simulink model "tut3"  (R2025b)
settings: Solver=VariableStepAuto  StartTime=0.0  StopTime=10.0  RelTol=1e-3
values from neighbouring files (symbols this model uses):
  A = [0 1 0 0 ... (first row only)    [untitled2.m]    (also in untitled3.m)
  A_hat = A_bb - Ke*A_ab    [untitled2.m]
  Aref = 0.8    [untitled3.m]
  B = [0; 0; 0; 1/m2]    [untitled2.m]    (also in untitled3.m = [0;1/m1;0;0])
  B_hat = A_hat*Ke + A_ba - Ke*A_aa    [untitled2.m]
  c1 = 2    [untitled2.m]    (also in untitled3.m)
  c2 = 5    [untitled2.m]    (also in untitled3.m)
  C_hat = [zeros(1, 3) ... (first row only)    [untitled2.m]
  D_hat = [1 ... (first row only)    [untitled2.m]
  F_hat = B_b - Ke*B_a    [untitled2.m]
  k1 = 4    [untitled2.m]    (also in untitled3.m)
  k2 = 12    [untitled2.m]    (also in untitled3.m)
  Kd = 35    [untitled3.m]
  Ke = place(A_bb', A_ab', p_o)'    [untitled2.m]
  Ki = 10    [untitled3.m]
  Kp = 120    [untitled3.m]
  m1 = 3    [untitled2.m]    (also in untitled3.m)
  w = 2*pi*1    (= 6.28318530718)    [untitled3.m]
  z0 = [2; 1.5; 1]    [untitled2.m]
settings Model: Creator=Abhi  LastModifiedBy=Abhi

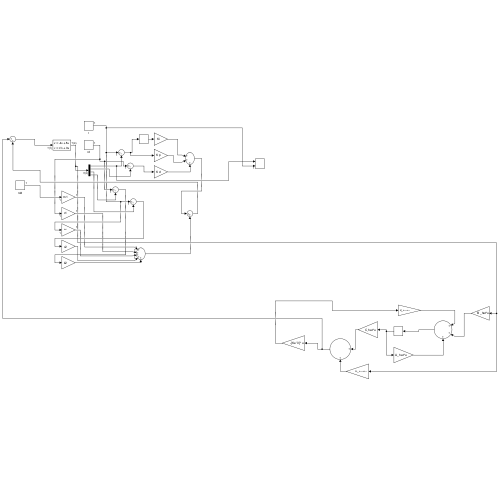
[thumbnail: Simulink's stored preview of the top-level diagram]
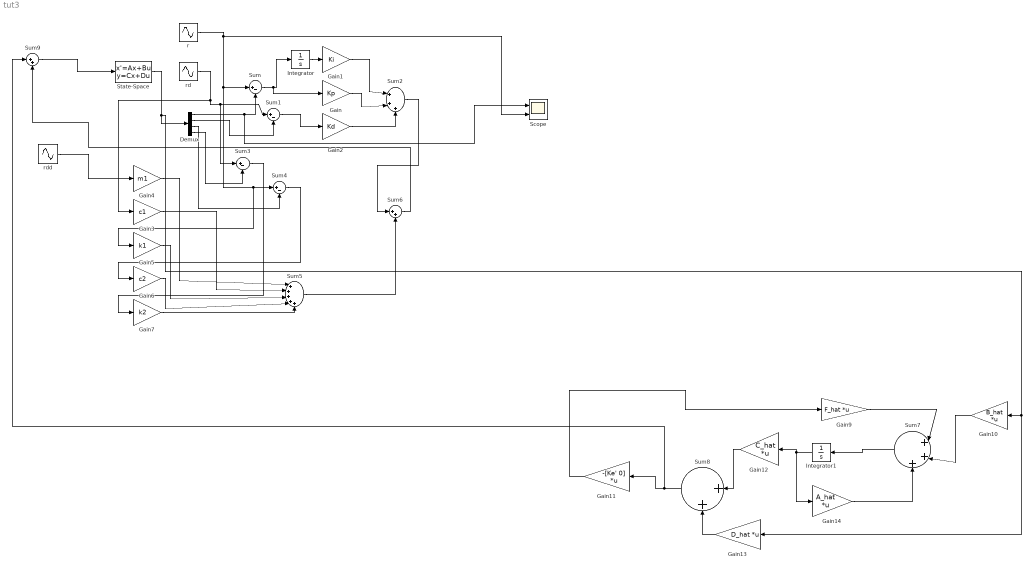
== system tut3 ==
  Demux : Demux
  Gain : Gain  Gain=Kp
  Gain1 : Gain  Gain=Ki
  Gain10 : Gain  Gain=B_hat  Multiplication=Matrix(K*u)
  Gain11 : Gain  Gain=-[Ke' 0]  Multiplication=Matrix(K*u)
  Gain12 : Gain  Gain=C_hat  Multiplication=Matrix(K*u)
  Gain13 : Gain  Gain=D_hat  Multiplication=Matrix(K*u)
  Gain14 : Gain  Gain=A_hat  Multiplication=Matrix(K*u)
  Gain2 : Gain  Gain=Kd
  Gain3 : Gain  Gain=c1
  Gain4 : Gain  Gain=m1
  Gain5 : Gain  Gain=k1
  Gain6 : Gain  Gain=c2
  Gain7 : Gain  Gain=k2
  Gain9 : Gain  Gain=F_hat  Multiplication=Matrix(K*u)
  Integrator : Integrator
  Integrator1 : Integrator  InitialCondition=z0
  Scope : Scope  NumInputPorts=2
      settings: ActiveDisplayYMinimum=-1.16819116268996  ActiveDisplayYMaximum=1.1667330676781473
  State-Space : StateSpace  A=A  B=B  C=eye(4)  D=zeros(4,1)  InitialCondition=[0.3 0.01 0 0]'
  Sum{,1,3..4} (4 alike) : Sum  Inputs=|+-
  Sum2 : Sum  Inputs=|+++
  Sum5 : Sum  Inputs=|+++++
  Sum6 : Sum  Inputs=|++
  Sum7 : Sum  Inputs=|+++
  Sum8 : Sum  Inputs=|++
  Sum9 : Sum  Inputs=|++
  r : Sin  Amplitude=Aref  Frequency=w  SampleTime=0
  rd : Sin  Amplitude=Aref*w  Frequency=w  Phase=pi/2  SampleTime=0
  rdd : Sin  Amplitude=Aref*w*w  Frequency=w  Phase=pi  SampleTime=0
  wires:
  Demux/1 -> Scope/1, Sum/2
  r/1 -> Scope/2, Gain5/1, Sum4/1, Sum/1
  Sum/1 -> Gain/1, Integrator/1
  Demux/2 -> Sum1/2
  rd/1 -> Gain3/1, Sum3/1, Sum1/1
  Integrator/1 -> Gain1/1
  Sum1/1 -> Gain2/1
  Gain1/1 -> Sum2/1
  Gain/1 -> Sum2/2
  Gain2/1 -> Sum2/3
  Demux/4 -> Sum3/2
  Demux/3 -> Sum4/2
  rdd/1 -> Gain4/1
  Sum3/1 -> Gain7/1
  Sum4/1 -> Gain6/1
  Gain4/1 -> Sum5/1
  Gain3/1 -> Sum5/2
  Gain5/1 -> Sum5/3
  Gain6/1 -> Sum5/4
  Gain7/1 -> Sum5/5
  Sum2/1 -> Sum6/1
  Sum5/1 -> Sum6/2
  Sum6/1 -> Sum9/2
  State-Space/1 -> Gain10/1, Gain13/1, Demux/1
  Sum8/1 -> Sum9/1, Gain11/1
  Gain11/1 -> Gain9/1
  Integrator1/1 -> Gain12/1, Gain14/1
  Gain12/1 -> Sum8/1
  Gain14/1 -> Sum7/3
  Gain10/1 -> Sum7/2
  Gain13/1 -> Sum8/2
  Gain9/1 -> Sum7/1
  Sum7/1 -> Integrator1/1
  Sum9/1 -> State-Space/1
